simulink model "Motor"  (R2025b)
settings: Solver=VariableStepAuto  StartTime=0.0  StopTime=10.0  RelTol=1e-3
libraries: autolibpmsminterior x1
settings Model: Creator=pc  LastModifiedBy=pc

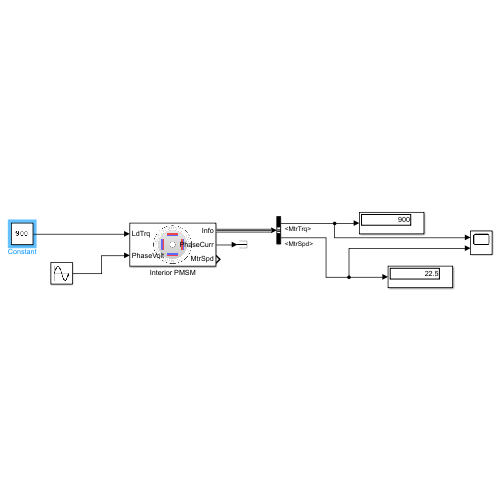
[thumbnail: Simulink's stored preview of the top-level diagram]
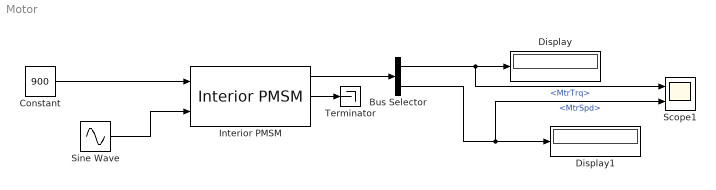
== system Motor ==
  Bus Selector : BusSelector  OutputSignals=MtrTrq,MtrSpd
  Constant : Constant  Value=900
  Display : Display
  Display1 : Display
  Interior PMSM : autolibpmsminterior/Interior PMSM  port_config=Torque  sim_type=Discrete  Ts=25e-6  P=4  Rs=0.008  Ldq=[0.00015, 0.00015]  KConstText=Permanent flux linkage constant (lambda_pm):  lambda_pm=0.12  Ke=159.9771  mechanical=[0.08, 0, 0]  idq0=[0 0]  theta_init=0  omega_init=0  KConst=0.2205  lambda_pm_calc=0.2205  Kt=0.07  RefBlkName='autolibpmsminterior/Interior PMSM'  aMode=5
      settings: LibrarySourceBlock=mcblib/Electrical Systems/Motors/Interior PMSM
  Scope1 : Scope  NumInputPorts=2
      settings: ActiveDisplayYMinimum=-18.286695629117879  ActiveDisplayYMaximum=67.16514409158286
  Sine Wave : Sin  Amplitude=50  Frequency=90  Phase=[0, -2*pi/3, -4*pi/3]  SampleTime=0
  Terminator : Terminator
  wires:
  Constant/1 -> Interior PMSM/1
  Sine Wave/1 -> Interior PMSM/2
  Interior PMSM/1 -> Bus Selector/1
  Interior PMSM/2 -> Terminator/1
  Bus Selector/1 -> Scope1/1, Display/1  "<MtrTrq>"
  Bus Selector/2 -> Scope1/2, Display1/1  "<MtrSpd>"
